simulink model "lvtest_table4"  (Simulink 7.1)
settings: Solver=ode4  StartTime=0.0  StopTime=1000  FixedStep=0.01  RelTol=1e-3
values from neighbouring files (symbols this model uses):
  c1 = 1.5    [find_bigvalue.m]    (also in find_bigvalue1.m)
  Ctorque = cq(2:5:102,2:5:182)    [lv_cankaofile.m]    (also in lv_demofile3.m)
  cut_in = 3    [lv_cankaofile.m]    (also in lv_demofile.m; lv_demofile1.m; lv_demofile2.m; lv_demofile3.m)
  cut_out = 25    [lv_cankaofile.m]    (also in lv_demofile.m; lv_demofile1.m; lv_demofile2.m; lv_demofile3.m)
  Jem = 90    [lv_cankaofile.m]    (also in lv_demofile.m = 97.5; lv_demofile1.m = 97.5; lv_demofile2.m = 97.5; lv_demofile3.m = 97.5)
  Jwt = 9e7    (= 90000000)    [lv_cankaofile.m]    (also in lv_demofile.m = 3275300; lv_demofile1.m = 3275300; lv_demofile2.m = 3275300; lv_demofile3.m = 3275300)
  K = 83    [lv_cankaofile.m]    (also in lv_demofile.m; lv_demofile1.m = 75.76; lv_demofile2.m; lv_demofile3.m = 75.76)
  R = 40    [lv_cankaofile.m]    (also in lv_demofile.m = 38.5; lv_demofile1.m = 38.75; lv_demofile2.m = 38.5; lv_demofile3.m = 38.5)
  ro_air = 1.225    [lv_cankaofile.m]    (also in lv_demofile.m = 1.2236; lv_demofile1.m; lv_demofile2.m = 1.2236; lv_demofile3.m)
  roughness = 600    [lv_cankaofile.m]    (also in lv_demofile1.m; lv_demofile3.m; lv_demofile4.m; lv_demofile5.m)
  steptime = 0.01    [lv_cankaofile.m]    (also in lv_demofile1.m; lv_demofile3.m; lv_demofile4.m; lv_demofile5.m)
  Tact = 0    [lv_cankaofile.m]    (also in lv_demofile.m; lv_demofile1.m; lv_demofile2.m; lv_demofile3.m)
  turb_int = 12    [lv_cankaofile.m]    (also in lv_demofile1.m; lv_demofile3.m; lv_demofile4.m; lv_demofile5.m)
  Ve = 13.5    [lv_cankaofile.m]    (also in lv_demofile1.m = 13; lv_demofile3.m; lv_demofile4.m = 13; lv_demofile5.m = 13)
undefined symbols (not defined in the file or in its folder): c2, c3, c4, c5, c6, u0
settings Model: Creator=xc  LastModifiedBy=lv

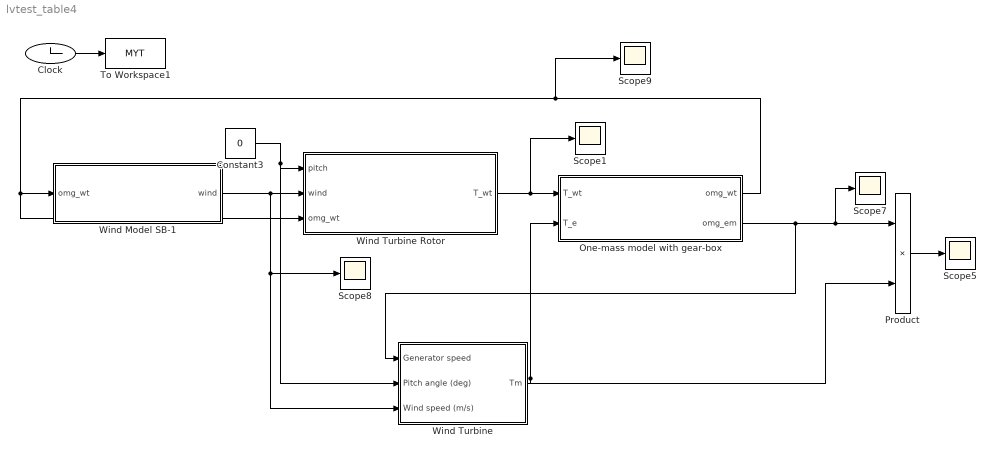
== system lvtest_table4 ==
  Clock : Clock
      settings: Decimation=10
  Constant3 : Constant  Value=0  OutDataType=sfix(16)  OutScaling=2^0
  One-mass model with gear-box : Subsystem  AncestorBlock=wt_blockset_v3/Mechanical Components/One-mass model with gear-box  mask(Simple Gearbox){Jem=Jem, Jwt=Jwt, K=K, init_speed=1.514}
      mask prompts: Jem "Electric machinery - Moment of inertia [kg m2]"; Jwt "Wind turbine rotor - Moment of inertia [kg*m2]"; K "Gearbox ratio"; init_speed "Initial condition [omg_wt (rad/sec)]"
      mask init:
      | J=Jem*K^2+Jwt;
      mask Display: disp('E M\nGear box')
  Product : Product  OutDataType=sfix(16)  OutScaling=2^0  RndMeth=Zero
  Scope{1,5,7..9} (5 alike) : Scope
      Scope1 settings: YMin=-150000  YMax=600000
      Scope5 settings: YMin=5000  YMax=40000  SaveName=ScopeData6
      Scope7 settings: TimeRange=100  YMin=-9000000  YMax=9000000  SaveName=ScopeData7
      Scope8 settings: YMin=-2.25e+010  YMax=1.5e+010  SaveName=ScopeData17
      Scope9 settings: SaveName=ScopeData8
  To Workspace1 : ToWorkspace  VariableName=MYT  SampleTime=-1  SaveFormat=Array
  Wind Model SB-1 : Subsystem  AncestorBlock=wt_blockset_v3/Mechanical Components/Wind Model SB-1  TreatAsAtomicUnit=on  mask(Wind Model using Simulink Band-limited white noise generator){D_rotor=2*R, v_mean=Ve, roughness=roughness, turb_int=turb_int, T_sample=steptime}
      mask prompts: D_rotor "Rotor diameter [m]"; v_mean "Average wind speed [m/sec]"; roughness "Length scale [m]"; turb_int "Turbulence intensity [%]"; T_sample "Sample time [sec]"
      mask help:
      | Implements a rotor wind model developped by RISOE National Laboratory based on Kaimal spectra. The model takes into account the rotational turbulences and the tower shadow.
      | This model uses the built-in band-limited white noise generator from Simulink with different seeds.
      mask init:
      | r = D_rotor/2;
      | sigma = v_mean*turb_int/100;
      | var = sigma^2;
      | c = roughness/(2*pi*v_mean);
      | d = r/v_mean;
      | trans=sigma*sqrt(roughness/v_mean);
      | random=[256, 894, 31];
      mask Display: disp('Wind\nModel\n(SB-1)')
  Wind Turbine : Subsystem  AncestorBlock=DRlib/Wind Generation/Wind Turbine  DialogController=POWERSYS.PowerSysDialog  mask(Wind Turbine){Pnom=1.5e6, Pelec_base=1.5e6/0.9, wind_base=12, P_wind_base=0.73, speed_nom=1.2, pitch_angle=0, DisplayTurbChar=off, c1_c6=[0.51763          116          0.4            5           21     0.006795], cp_nom=0.48, lambda_nom=8.1}
      mask prompts: Pnom "Nominal mechanical output power (W):"; Pelec_base "Base power of the electrical generator (VA):"; wind_base "Base wind speed (m/s):"; P_wind_base "Maximum power at base wind speed (pu of nominal mechanical power):"; speed_nom "Base rotational speed (p.u. of base generator speed):"; pitch_angle "Pitch angle beta to display wind-turbine power characteristics (beta >=0)  (deg):"; DisplayTurbChar "Display wind turbine power characteristics"
      mask help:
      | This block implements a variable pitch wind turbine model. The performance coefficient Cp of the turbine is the mechanical output power of the turbine divided by wind power and a function of wind speed, rotational speed, and pitch angle (beta). Cp reaches its maximum value at zero beta. Select the wind-turbine power characteristics display to plot the turbine characteristics at the specified pitch angle.
      |
      | The first input is the generator speed in per unit of the generator base speed. For a synchronous or asynchronous generator, the base speed is the synchronous speed. For a permanent-magnet generator, the base speed is defined as the speed producing nominal voltage at  no load. The second input is the blade pitch angle (beta) in degrees. The third input is the wind speed in m/s.
      |
      | The output is the torque applied to the generator shaft in per unit of the generator ratings.
      |
      | The turbine inertia must be added to the generator inertia.
      mask init:
      | %Wind turbine typical characteristic data
      | %c2=116;c3=0.4;c4=5;c5=21;
      | %Computation of c1 and c6 for lambda_nom et cpmax
      | %lambda_nom=8.1;
      | %cp_max=0.48;
      | %cp_nom=cp_max;
      | 
      | %lambda_i_nom=1/(1/lambda_nom-0.035);
      | %k_nom=-(c2*c5/lambda_i_nom-c4*c5-c2)*exp(-c5/lambda_i_nom)/lambda_nom^2;
      | %c1=cp_max/((c2/lambda_i_nom-c4)*exp(-c5/lambda_i_nom)+k_nom*lambda_nom);
      | %c6=k_nom*c1;
      | power_initmask();
      mask Help: web(psbhelp);
      mask CallbackString:
      | ParVisible={'on','on','on','on','on','on','on','off','off','off',};
      | set_param(gcb,'MaskVisibilities',ParVisible);
      | c1_c6=str2num(get_param(gcb,'c1_c6'));
      | c1=c1_c6(1);c2=c1_c6(2);c3=c1_c6(3);c4=c1_c6(4);c5=c1_c6(5);c6=c1_c6(6);||||||DisplayTurbChar=get_param(gcb,'DisplayTurbChar');
      | 
      | if strcmp(DisplayTurbChar,'on')
      |     fig_num=figure;
      | 	clf(fig_num);
      | 	[speed_nom,wind_base,P_wind_base,pitch_angle]=getSPSmaskvalues(gcb,{'speed_nom','wind_base','P_wind_base','pitch_angle'});
      | 	[c1_c6,lambda_nom,cp_nom]=getSPSmaskvalues(gcb,{'c1_c6','lambda_nom','cp_nom'});
      | 	c1=c1_c6(1);c2=c1_c6(2);c3=c1_c6(3);c4=c1_c6(4);c5=c1_c6(5);c6=c1_c6(6);
      | 
      | 	%Wind turbine typical characteristic data
      |     %c2=116;c3=0.4;c4=5;c5=21;
      |     %Computation of c1 and c6 for lambda_nom et cpmax
      |     %lambda_nom=8.1;
      |     %cp_max=0.48;
      |     %cp_nom=cp_max;
      | 
      |     %lambda_i_nom=1/(1/lambda_nom-0.035);
      |     %k_nom=-(c2*c5/lambda_i_nom-c4*c5-c2)*exp(-c5/lambda_i_nom)/lambda_nom^2;
      |     %c1=cp_max/((c2/lambda_i_nom-c4)*exp(-c5/lambda_i_nom)+k_nom*lambda_nom);
      |     %c6=k_nom*c1;
      | 
      | 	wr_elec_pu=1e-3:0.01:1.5;;
      |     wr_mec_pu=wr_elec_pu/speed_nom;
      |     wind_max=ceil((1.2/P_wind_base)^(1/3)*wind_base);
      |     wind_min=round(((0.1)/P_wind_base)^(1/3)*wind_base);
      |     wind1=wind_min:(wind_base-wind_min)/5:wind_base;
      |     wind2=wind_base+(wind_base-wind_min)/5:(wind_base-wind_min)/5:wind_max;
      |     wind_pu=[wind1 wind2]/wind_base;
      | 
      |     for k=1:length(wind_pu)
      |         for i=1:length(wr_mec_pu);
      |             lambda_pu=wr_mec_pu(i)/wind_pu(k);
      |             lambda=lambda_pu*lambda_nom;
      |             lambda_i=1/(1/(lambda+0.08*pitch_angle)-0.035/(pitch_angle^3+1));
      |             cp=c1*(c2/lambda_i-c3*pitch_angle-c4)*exp(-c5/lambda_i)+c6*lambda;
      |             cp_pu=cp/cp_nom;
      |             Pwind_pu(k,i)=wind_pu(k)^3*cp_pu*P_wind_base;
      |         end
      |     end
      |     for k=1:length(wind_pu)
      |         plot(wr_elec_pu,Pwind_pu(k,:))
      |         hold on
      |     end
      | 
      |     plot([speed_nom,speed_nom,0],[0,P_wind_base,P_wind_base],'r--')
      |     text(speed_nom+0.01,0+0.05,sprintf('%0.4g pu',speed_nom))
      |     text(0.01,P_wind_base+0.05,sprintf('Max. power at base wind speed (%0.4g m/s) and beta = 0 deg',wind_base))
      |     for i=1:length(wind_pu),
      |         p_max(i)=max(Pwind_pu(i,:));
      |         speed(i)=wr_elec_pu(find(Pwind_pu(i,:)==p_max(i)));
      |         text(speed(i),p_max(i),sprintf('%0.4g m/s',wind_pu(i)*wind_base))
      |     end
      |     plot([0 max(wr_elec_pu)],[0 0],'--')
      | 
      |     xlabel('Turbine speed (pu of nominal generator speed)')
      |     ylabel('Turbine output power (pu of nominal mechanical power)')
      |     title(sprintf('Turbine Power Characteristics (Pitch angle beta = %0.4g deg)',pitch_angle))
      |     axis([0 max(wr_elec_pu) min(Pwind_pu(1,:)) max(P_wind_base+0.1,max(wind_pu)^3*P_wind_base+0.1)])
      |     set_param(gcb,'DisplayTurbChar','off')
      | end|||
      mask Display: disp('');
  Wind Turbine Rotor : Subsystem  AncestorBlock=wt_blockset_beta/Mechanical Components/Wind Turbine Rotor  mask(Aerodynamic model for wind turbine){R=R, ro_air=ro_air, cut_in=cut_in, cut_out=cut_out, Tact=Tact}
      mask prompts: R "Blade radius [m]"; ro_air "Air density [kg m3]"; cut_in "Cut in speed [m/sec]"; cut_out "Cut out speed [m/sec]"; Tact "Time constant for pitch actuator [sec]"
      mask init:
      | %cq_table
      mask Display: plot(20,0,120,200,[45,35,35,45,75,75,45],[85,92,108,115,115,85,85],[55,50,70,65],[115,180,190,115],[55,50,70,65],[85,10,20,85],[75,85],[102,102],[75,85],[98,98],[105,85,85,105],[80,85,115,120])
  wires:
  Wind Turbine Rotor/1(T_wt) -> One-mass model with gear-box/1(T_wt), Scope1/1
  Constant3/1 -> Wind Turbine Rotor/1(pitch), Wind Turbine/2(Pitch angle (deg))
  Wind Model SB-1/1(wind) -> Wind Turbine Rotor/2(wind), Scope8/1, Wind Turbine/3(Wind speed (m/s))
  One-mass model with gear-box/1(omg_wt) -> Scope9/1, Wind Turbine Rotor/3(omg_wt), Wind Model SB-1/1(omg_wt)
  One-mass model with gear-box/2(omg_em) -> Product/1, Scope7/1, Wind Turbine/1("Generator speed ")
  Clock/1 -> To Workspace1/1
  Product/1 -> Scope5/1
  Wind Turbine/1("Tm ") -> One-mass model with gear-box/2(T_e), Product/2

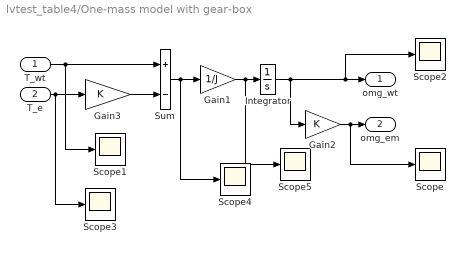
== system lvtest_table4/One-mass model with gear-box ==
  T_wt : Inport  OutDataType=sfix(16)  OutScaling=2^0
  T_e : Inport  Port=2  OutDataType=sfix(16)  OutScaling=2^0
  Gain1 : Gain  Gain=1/J  ParameterDataType=sfix(16)  ParameterScaling=2^0  OutDataType=sfix(16)  OutScaling=2^0  SaturateOnIntegerOverflow=on  OutDataTypeStr=Inherit: Same as input  ParamDataTypeStr=Inherit: Same as input
  Gain2 : Gain  Gain=K  ParameterDataType=sfix(16)  ParameterScaling=2^0  OutDataType=sfix(16)  OutScaling=2^0  SaturateOnIntegerOverflow=on  OutDataTypeStr=Inherit: Same as input  ParamDataTypeStr=Inherit: Same as input
  Gain3 : Gain  Gain=K  ParameterDataType=sfix(16)  ParameterScaling=2^0  OutDataType=sfix(16)  OutScaling=2^0  SaturateOnIntegerOverflow=on  OutDataTypeStr=Inherit: Same as input  ParamDataTypeStr=Inherit: Same as input
  Integrator : Integrator  InitialCondition=init_speed  UpperSaturationLimit=0.95*2*pi*60  LowerSaturationLimit=0
  Scope{,1..5} (6 alike) : Scope
      Scope settings: TimeRange=10  SaveName=ScopeData20
      Scope1 settings: TimeRange=10  SaveName=ScopeData24
      Scope2 settings: YMin=-2.25e+010  YMax=1.5e+010  SaveName=ScopeData21
      Scope3 settings: TimeRange=10  SaveName=ScopeData25
      Scope4 settings: TimeRange=10  SaveName=ScopeData2
      Scope5 settings: TimeRange=10  SaveName=ScopeData22
  Sum : Sum  Inputs=+-  OutDataType=sfix(16)  OutScaling=2^0  SaturateOnIntegerOverflow=on  InputSameDT=on  OutDataTypeStr=Inherit: Same as first input
  omg_wt : Outport  OutDataType=sfix(16)  OutScaling=2^0  InitialOutput=0
  omg_em : Outport  Port=2  OutDataType=sfix(16)  OutScaling=2^0  InitialOutput=0
  wires:
  Gain3/1 -> Sum/2
  Gain2/1 -> omg_em/1, Scope/1
  Integrator/1 -> Gain2/1, omg_wt/1, Scope2/1
  T_wt/1 -> Sum/1, Scope1/1
  T_e/1 -> Gain3/1, Scope3/1
  Sum/1 -> Gain1/1, Scope4/1
  Gain1/1 -> Integrator/1, Scope5/1

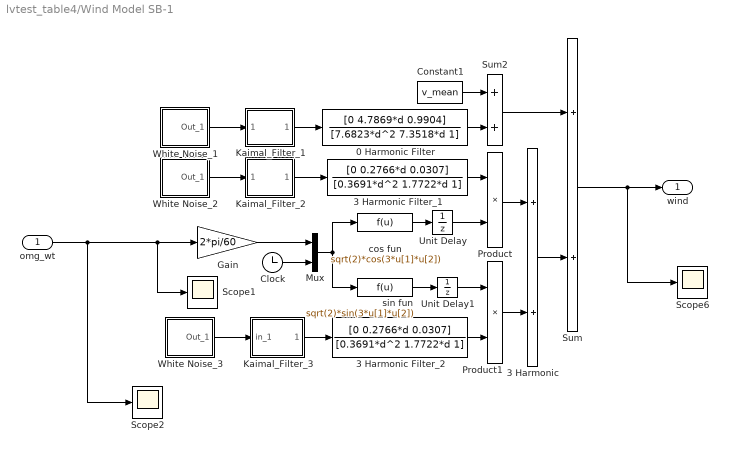
== system lvtest_table4/Wind Model SB-1 ==
  omg_wt : Inport  OutDataType=sfix(16)  OutScaling=2^0
  0 Harmonic Filter : TransferFcn  Numerator=[0 4.7869*d 0.9904]  Denominator=[7.6823*d^2 7.3518*d 1]
  3 Harmonic : Sum  OutDataType=sfix(16)  OutScaling=2^0  SaturateOnIntegerOverflow=on  InputSameDT=on  OutDataTypeStr=Inherit: Same as first input
  3 Harmonic Filter_1 : TransferFcn  Numerator=[0 0.2766*d 0.0307]  Denominator=[0.3691*d^2 1.7722*d 1]
  3 Harmonic Filter_2 : TransferFcn  Numerator=[0 0.2766*d 0.0307]  Denominator=[0.3691*d^2 1.7722*d 1]
  Clock : Clock
  Constant1 : Constant  Value=v_mean  OutDataType=sfix(16)  OutScaling=2^0
  Gain : Gain  Gain=2*pi/60  ParameterDataType=sfix(16)  ParameterScaling=2^0  OutDataType=sfix(16)  OutScaling=2^0  SaturateOnIntegerOverflow=on  OutDataTypeStr=Inherit: Same as input  ParamDataTypeStr=Inherit: Same as input
  Kaimal_Filter_1 : Subsystem
  Kaimal_Filter_2 : Subsystem
  Kaimal_Filter_3 : Subsystem
  Mux : Mux  Inputs=2
  Product : Product  OutDataType=sfix(16)  OutScaling=2^0  SaturateOnIntegerOverflow=on  InputSameDT=on  OutDataTypeStr=Inherit: Same as first input
  Product1 : Product  OutDataType=sfix(16)  OutScaling=2^0  SaturateOnIntegerOverflow=on  InputSameDT=on  OutDataTypeStr=Inherit: Same as first input
  Scope1 : Scope
      settings: YMin=-2.25e+010  YMax=1.5e+010  SaveName=ScopeData22
  Scope2 : Scope
      settings: YMin=-2.25e+010  YMax=1.5e+010  SaveName=ScopeData20
  Scope6 : Scope
      settings: TimeRange=100  YMin=-9e+006  YMax=9e+006  SaveName=ScopeData39
  Sum : Sum  OutDataType=sfix(16)  OutScaling=2^0  SaturateOnIntegerOverflow=on  InputSameDT=on  OutDataTypeStr=Inherit: Same as first input
  Sum2 : Sum  OutDataType=sfix(16)  OutScaling=2^0  SaturateOnIntegerOverflow=on  InputSameDT=on  OutDataTypeStr=Inherit: Same as first input
  Unit Delay : UnitDelay  SampleTime=T_sample
  Unit Delay1 : UnitDelay  SampleTime=T_sample
  White Noise_1 : Subsystem  mask(Continuous White Noise.){Cov=[1], Ts=T_sample, seed=[random(1)]}
      mask prompts: Cov "Noise Power:"; Ts "Sample Time:"
      mask help:
      | White noise for continuous (s-domain) systems.
      | Band-limited using zero-order-hold.
      mask init:
      | r = rand(1,12); r2 = [r(1),r;r,r(12)]; t =[1:13;1:13];
      mask Help: Implemented using white noise into Zero-Order Hold block. The seed and power can be vectors of the same length to produce a vector of white noise sources. For faster simulation, set sample time to the highest value possible but in accordance with the fastest dynamics of system.
      mask Display: plot(t(:),r2(:))
  White Noise_2 : Subsystem  mask(Continuous White Noise.){@1=[1], @2=T_sample, @3=[random(2)]}
      mask prompts: @1 "Noise Power:"; @2 "Sample Time:"; @3 "Seed"
      mask help:
      | White noise for continuous (s-domain) systems.
      | Band-limited using zero-order-hold.
      mask init:
      | Cov = @1; Ts = @2; seed = @3; r = rand(1,12); r2 = [r(1),r;r,r(12)]; t =[1:13;1:13];
      mask Help: Implemented using white noise into Zero-Order Hold block. The seed and power can be vectors of the same length to produce a vector of white noise sources. For faster simulation, set sample time to the highest value possible but in accordance with the fastest dynamics of system.
      mask Display: plot(t(:),r2(:))
  White Noise_3 : Subsystem  mask(Continuous White Noise.){@1=[1], @2=T_sample, @3=[random(3)]}
      mask prompts: @1 "Noise Power:"; @2 "Sample Time:"; @3 "Seed"
      mask help:
      | White noise for continuous (s-domain) systems.
      | Band-limited using zero-order-hold.
      mask init:
      | Cov = @1; Ts = @2; seed = @3; r = rand(1,12); r2 = [r(1),r;r,r(12)]; t =[1:13;1:13];
      mask Help: Implemented using white noise into Zero-Order Hold block. The seed and power can be vectors of the same length to produce a vector of white noise sources. For faster simulation, set sample time to the highest value possible but in accordance with the fastest dynamics of system.
      mask Display: plot(t(:),r2(:))
  cos fun : Fcn  Expr=sqrt(2)*cos(3*u[1]*u[2])
  sin fun : Fcn  Expr=sqrt(2)*sin(3*u[1]*u[2])
  wind : Outport  OutDataType=sfix(16)  OutScaling=2^0  InitialOutput=[u0]
  wires:
  Clock/1 -> Mux/2
  Unit Delay1/1 -> Product1/1
  Unit Delay/1 -> Product/2
  Gain/1 -> Mux/1
  omg_wt/1 -> Gain/1, Scope1/1, Scope2/1
  Mux/1 -> sin fun/1, cos fun/1
  3 Harmonic Filter_1/1 -> Product/1
  White Noise_3/1(Out_1) -> Kaimal_Filter_3/1(in_1)
  White Noise_2/1(Out_1) -> Kaimal_Filter_2/1(in_1)
  White Noise_1/1(Out_1) -> Kaimal_Filter_1/1(in_1)
  Kaimal_Filter_1/1(out_1) -> 0 Harmonic Filter/1
  Sum/1 -> wind/1, Scope6/1
  Constant1/1 -> Sum2/1
  Sum2/1 -> Sum/1
  0 Harmonic Filter/1 -> Sum2/2
  3 Harmonic/1 -> Sum/2
  3 Harmonic Filter_2/1 -> Product1/2
  Product1/1 -> 3 Harmonic/2
  Product/1 -> 3 Harmonic/1
  sin fun/1 -> Unit Delay1/1
  cos fun/1 -> Unit Delay/1
  Kaimal_Filter_3/1(out_1) -> 3 Harmonic Filter_2/1
  Kaimal_Filter_2/1(out_1) -> 3 Harmonic Filter_1/1

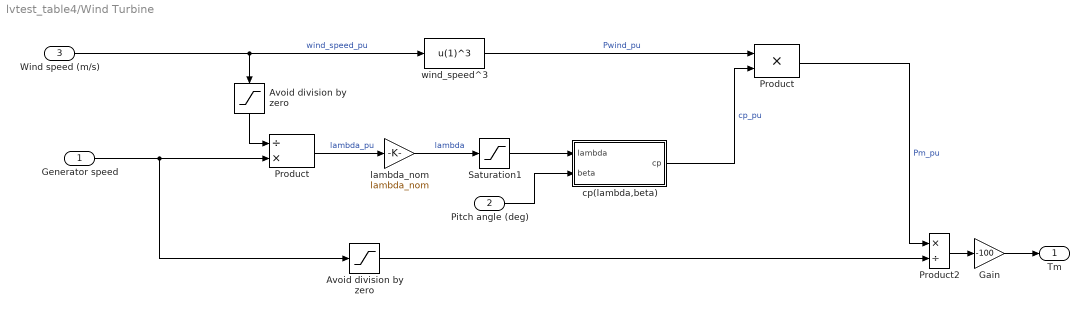
== system lvtest_table4/Wind Turbine ==
  "Generator speed " : Inport  OutDataType=sfix(16)  OutScaling=2^0
  Pitch angle (deg) : Inport  Port=2  OutDataType=sfix(16)  OutScaling=2^0
  Wind speed (m/s) : Inport  Port=3  OutDataType=sfix(16)  OutScaling=2^0
  Avoid division by zero : Saturate  UpperLimit=1e6  LowerLimit=1e-6  OutDataType=sfix(16)  OutScaling=2^0
  "Avoid division by zero " : Saturate  Orientation=down  UpperLimit=1e6  LowerLimit=1e-6  OutDataType=sfix(16)  OutScaling=2^0
  Gain : Gain  Gain=-100  ParameterDataType=sfix(16)  ParameterScaling=2^0  OutDataType=sfix(16)  OutScaling=2^0  SaturateOnIntegerOverflow=on  OutDataTypeStr=Inherit: Same as input  ParamDataTypeStr=Inherit: Same as input
  Product : Product  Inputs=/*  OutDataType=sfix(16)  OutScaling=2^0  SaturateOnIntegerOverflow=on  OutDataTypeStr=Inherit: Same as first input
  "Product " : Product  OutDataType=sfix(16)  OutScaling=2^0  SaturateOnIntegerOverflow=on  OutDataTypeStr=Inherit: Same as first input
  Product2 : Product  Inputs=*/  OutDataType=sfix(16)  OutScaling=2^0  SaturateOnIntegerOverflow=on  InputSameDT=on  OutDataTypeStr=Inherit: Same as first input
  Saturation1 : Saturate  UpperLimit=inf  LowerLimit=1e-6  OutDataType=sfix(16)  OutScaling=2^0
  cp(lambda,beta) : Subsystem
  lambda_nom : Gain  Gain=lambda_nom  ParameterDataType=sfix(16)  ParameterScaling=2^0  OutDataType=sfix(16)  OutScaling=2^0  SaturateOnIntegerOverflow=on  OutDataTypeStr=Inherit: Same as input  ParamDataTypeStr=Inherit: Same as input
  wind_speed^3 : Fcn  Expr=u(1)^3
  "Tm " : Outport  OutDataType=sfix(16)  OutScaling=2^0
  wires:
  "Avoid division by zero "/1 -> Product/1
  Product/1 -> lambda_nom/1  "lambda_pu"
  Saturation1/1 -> cp(lambda,beta)/1(lambda)
  cp(lambda,beta)/1(cp) -> "Product "/2  "cp_pu"
  lambda_nom/1 -> Saturation1/1  "lambda"
  "Product "/1 -> Product2/1  "Pm_pu"
  "Generator speed "/1 -> Avoid division by zero/1, Product/2
  Gain/1 -> "Tm "/1
  Wind speed (m/s)/1 -> "Avoid division by zero "/1, wind_speed^3/1  "wind_speed_pu"
  Avoid division by zero/1 -> Product2/2
  Product2/1 -> Gain/1
  wind_speed^3/1 -> "Product "/1  "Pwind_pu"
  Pitch angle (deg)/1 -> cp(lambda,beta)/2(beta)

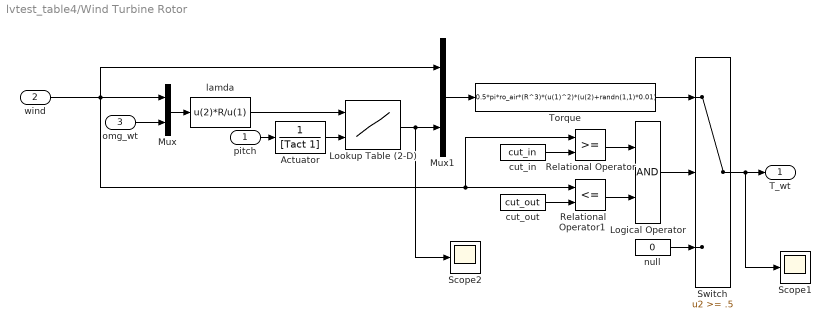
== system lvtest_table4/Wind Turbine Rotor ==
  pitch : Inport  OutDataType=sfix(16)  OutScaling=2^0
  wind : Inport  Port=2  OutDataType=sfix(16)  OutScaling=2^0
  omg_wt : Inport  Port=3  OutDataType=sfix(16)  OutScaling=2^0
  Actuator : TransferFcn  Denominator=[Tact 1]
  Logical Operator : Logic
  Lookup Table (2-D) : Lookup2D  RowIndex=[0:1:20]  ColumnIndex=[-90:5:90]  Table=Ctorque  OutDataType=sfix(16)  OutScaling=2^0
  Mux : Mux  Inputs=2
  Mux1 : Mux  Inputs=2
  Relational Operator : RelationalOperator  InputSameDT=on
  Relational Operator1 : RelationalOperator  Operator=<=  InputSameDT=on
  Scope1 : Scope
      settings: TimeRange=20  YMin=-1500000  YMax=1500000  SaveName=ScopeData19
  Scope2 : Scope
      settings: TimeRange=20  YMin=0.0025  YMax=0.0325  SaveName=ScopeData35
  Switch : Switch  Threshold=.5  SaturateOnIntegerOverflow=on  InputSameDT=on
  Torque : Fcn  Expr=0.5*pi*ro_air*(R^3)*(u(1)^2)*(u(2)+randn(1,1)*0.01)
  cut_in : Constant  Value=cut_in  OutDataType=sfix(16)  OutScaling=2^0
  cut_out : Constant  Value=cut_out  OutDataType=sfix(16)  OutScaling=2^0
  lamda : Fcn  Expr=u(2)*R/u(1)
  null : Constant  Value=0  OutDataType=sfix(16)  OutScaling=2^0
  T_wt : Outport
  wires:
  Actuator/1 -> Lookup Table (2-D)/2
  Mux/1 -> lamda/1
  Mux1/1 -> Torque/1
  omg_wt/1 -> Mux/2
  cut_in/1 -> Relational Operator/2
  cut_out/1 -> Relational Operator1/2
  Relational Operator1/1 -> Logical Operator/2
  Relational Operator/1 -> Logical Operator/1
  Switch/1 -> T_wt/1, Scope1/1
  Torque/1 -> Switch/1
  null/1 -> Switch/3
  Logical Operator/1 -> Switch/2
  wind/1 -> Mux/1, Relational Operator/1, Relational Operator1/1, Mux1/1
  Lookup Table (2-D)/1 -> Mux1/2, Scope2/1
  lamda/1 -> Lookup Table (2-D)/1
  pitch/1 -> Actuator/1

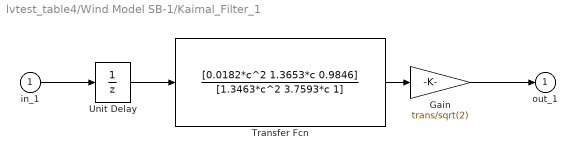
== system lvtest_table4/Wind Model SB-1/Kaimal_Filter_1 ==
  in_1 : Inport  OutDataType=sfix(16)  OutScaling=2^0
  Gain : Gain  Gain=trans/sqrt(2)  ParameterDataType=sfix(16)  ParameterScaling=2^0  OutDataType=sfix(16)  OutScaling=2^0  SaturateOnIntegerOverflow=on  OutDataTypeStr=Inherit: Same as input  ParamDataTypeStr=Inherit: Same as input
  Transfer Fcn : TransferFcn  Numerator=[0.0182*c^2 1.3653*c 0.9846]  Denominator=[1.3463*c^2 3.7593*c 1]
  Unit Delay : UnitDelay  SampleTime=T_sample
  out_1 : Outport  OutDataType=sfix(16)  OutScaling=2^0
  wires:
  Transfer Fcn/1 -> Gain/1
  in_1/1 -> Unit Delay/1
  Gain/1 -> out_1/1
  Unit Delay/1 -> Transfer Fcn/1

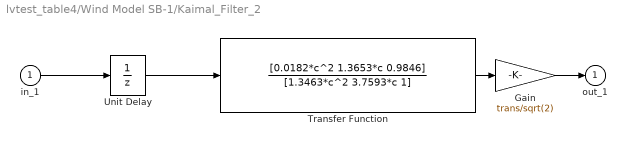
== system lvtest_table4/Wind Model SB-1/Kaimal_Filter_2 ==
  in_1 : Inport  OutDataType=sfix(16)  OutScaling=2^0
  Gain : Gain  Gain=trans/sqrt(2)  ParameterDataType=sfix(16)  ParameterScaling=2^0  OutDataType=sfix(16)  OutScaling=2^0  SaturateOnIntegerOverflow=on  OutDataTypeStr=Inherit: Same as input  ParamDataTypeStr=Inherit: Same as input
  Transfer Function : TransferFcn  Numerator=[0.0182*c^2 1.3653*c 0.9846]  Denominator=[1.3463*c^2 3.7593*c 1]
  Unit Delay : UnitDelay  SampleTime=T_sample
  out_1 : Outport  OutDataType=sfix(16)  OutScaling=2^0
  wires:
  Transfer Function/1 -> Gain/1
  in_1/1 -> Unit Delay/1
  Gain/1 -> out_1/1
  Unit Delay/1 -> Transfer Function/1

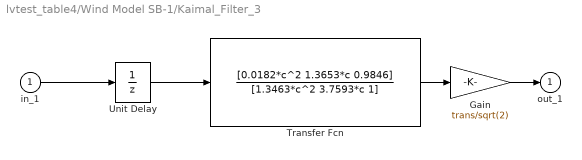
== system lvtest_table4/Wind Model SB-1/Kaimal_Filter_3 ==
  in_1 : Inport  OutDataType=sfix(16)  OutScaling=2^0
  Gain : Gain  Gain=trans/sqrt(2)  ParameterDataType=sfix(16)  ParameterScaling=2^0  OutDataType=sfix(16)  OutScaling=2^0  SaturateOnIntegerOverflow=on  OutDataTypeStr=Inherit: Same as input  ParamDataTypeStr=Inherit: Same as input
  Transfer Fcn : TransferFcn  Numerator=[0.0182*c^2 1.3653*c 0.9846]  Denominator=[1.3463*c^2 3.7593*c 1]
  Unit Delay : UnitDelay  SampleTime=T_sample
  out_1 : Outport  OutDataType=sfix(16)  OutScaling=2^0
  wires:
  Transfer Fcn/1 -> Gain/1
  in_1/1 -> Unit Delay/1
  Gain/1 -> out_1/1
  Unit Delay/1 -> Transfer Fcn/1

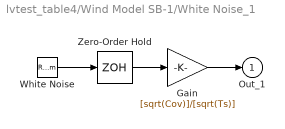
== system lvtest_table4/Wind Model SB-1/White Noise_1 ==
  Gain : Gain  Gain=[sqrt(Cov)]/[sqrt(Ts)]  ParameterDataType=sfix(16)  ParameterScaling=2^0  OutDataType=sfix(16)  OutScaling=2^0  SaturateOnIntegerOverflow=on  OutDataTypeStr=Inherit: Same as input  ParamDataTypeStr=Inherit: Same as input
  White Noise : RandomNumber  Seed=seed  SampleTime=Ts
  Zero-Order Hold : ZeroOrderHold  SampleTime=Ts
  Out_1 : Outport  OutDataType=sfix(16)  OutScaling=2^0
  wires:
  Zero-Order Hold/1 -> Gain/1
  Gain/1 -> Out_1/1
  White Noise/1 -> Zero-Order Hold/1

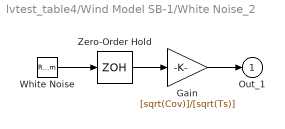
== system lvtest_table4/Wind Model SB-1/White Noise_2 ==
  Gain : Gain  Gain=[sqrt(Cov)]/[sqrt(Ts)]  ParameterDataType=sfix(16)  ParameterScaling=2^0  OutDataType=sfix(16)  OutScaling=2^0  SaturateOnIntegerOverflow=on  OutDataTypeStr=Inherit: Same as input  ParamDataTypeStr=Inherit: Same as input
  White Noise : RandomNumber  Seed=seed  SampleTime=Ts
  Zero-Order Hold : ZeroOrderHold  SampleTime=Ts
  Out_1 : Outport  OutDataType=sfix(16)  OutScaling=2^0
  wires:
  Zero-Order Hold/1 -> Gain/1
  Gain/1 -> Out_1/1
  White Noise/1 -> Zero-Order Hold/1

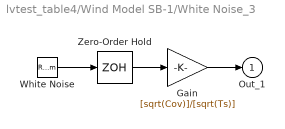
== system lvtest_table4/Wind Model SB-1/White Noise_3 ==
  Gain : Gain  Gain=[sqrt(Cov)]/[sqrt(Ts)]  ParameterDataType=sfix(16)  ParameterScaling=2^0  OutDataType=sfix(16)  OutScaling=2^0  SaturateOnIntegerOverflow=on  OutDataTypeStr=Inherit: Same as input  ParamDataTypeStr=Inherit: Same as input
  White Noise : RandomNumber  Seed=seed  SampleTime=Ts
  Zero-Order Hold : ZeroOrderHold  SampleTime=Ts
  Out_1 : Outport  OutDataType=sfix(16)  OutScaling=2^0
  wires:
  Zero-Order Hold/1 -> Gain/1
  Gain/1 -> Out_1/1
  White Noise/1 -> Zero-Order Hold/1

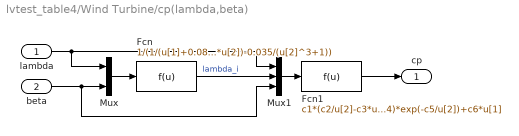
== system lvtest_table4/Wind Turbine/cp(lambda,beta) ==
  lambda : Inport  OutDataType=sfix(16)  OutScaling=2^0
  beta : Inport  Port=2  OutDataType=sfix(16)  OutScaling=2^0
  Fcn : Fcn  Expr=1/(1/(u[1]+0.08*u[2])-0.035/(u[2]^3+1))
  Fcn1 : Fcn  Expr=c1*(c2/u[2]-c3*u[3]-c4)*exp(-c5/u[2])+c6*u[1]
  Mux : Mux  Inputs=2
  Mux1 : Mux  Inputs=3
  cp : Outport  OutDataType=sfix(16)  OutScaling=2^0
  wires:
  Mux/1 -> Fcn/1
  beta/1 -> Mux/2, Mux1/3
  Mux1/1 -> Fcn1/1
  lambda/1 -> Mux/1, Mux1/1
  Fcn1/1 -> cp/1
  Fcn/1 -> Mux1/2  "lambda_i"
